simulink model "KALTITUDE_V1"  (R2015b)
settings: Solver=ode2  StartTime=0.0  StopTime=65  FixedStep=0.01  RelTol=1e-3
undefined symbols (not defined in the file or in its folder): sigbuilder_block
settings Model: SimulationMode=accelerator  Creator=asus  LastModifiedBy=asus

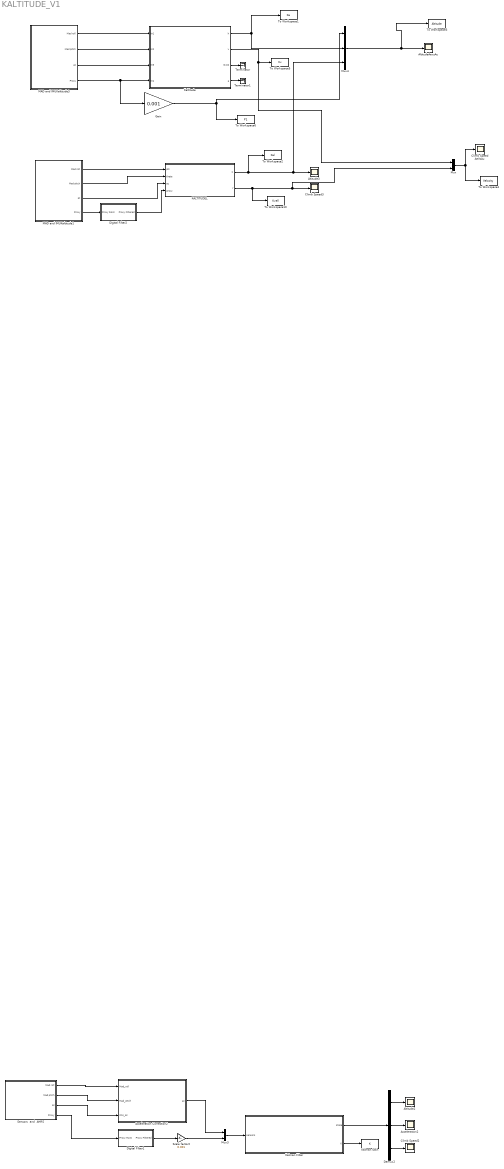
== system KALTITUDE_V1 ==
  Acceleration Correction2 : MATLAB Function  TreatAsAtomicUnit=on
  Acceleration2 : Scope
  Altitude2 : Scope
  Altitude3 : Scope
  AltitudeAevsAu : Scope
  Climb Speed AeVsAu : Scope
  Climb Speed2 : Scope
  Climb Speed3 : Scope
  Demux2 : Demux  Outputs=[1 1 1]
  Digital Filter1 : Subsystem
  Digital Filter2 : Subsystem
  Gain : Gain  Gain=0.001
  KALTITUDEL : Subsystem
  Kalman Filter : Subsystem
  Kalman Gain : ToWorkspace  VariableName=K  SaveFormat=Timeseries  SampleTime=-1
  Kaltitude : Subsystem
  MAD and IMUKaltitude1 : Subsystem
  MAD and IMUKaltitude3 : Subsystem
  Mux : Mux  Inputs=[1 1]
  Mux3 : Mux  Inputs=2
  Mux4 : Mux  Inputs=[1 1 1]
  Scale factor2 : Gain  Gain=0.001
  "Sensors  and  AHRS " : Subsystem
  Terminator : Terminator
  Terminator1 : Terminator
  To Workspace1 : ToWorkspace  VariableName=Ka  SampleTime=-1
  To Workspace10 : ToWorkspace  VariableName=Kvell  SampleTime=-1
  To Workspace2 : ToWorkspace  VariableName=Kal  SampleTime=-1
  To Workspace3 : ToWorkspace  VariableName=Altitude  SampleTime=-1
  To Workspace4 : ToWorkspace  VariableName=Velocity  SampleTime=-1
  To Workspace5 : ToWorkspace  VariableName=Kv  SampleTime=-1
  To Workspace6 : ToWorkspace  VariableName=P1  SampleTime=-1
  wires:
  Kalman Filter/1(state) -> Demux2/1
  Kalman Filter/2(K) -> Kalman Gain/1
  Mux3/1 -> Kalman Filter/1(sensors)
  Demux2/1 -> Altitude2/1
  Demux2/3 -> Climb Speed2/1
  Demux2/2 -> Acceleration2/1
  Scale factor2/1 -> Mux3/2
  Acceleration Correction2/1(az) -> Mux3/1
  "Sensors  and  AHRS "/1(Mad roll) -> Acceleration Correction2/1(Mad_roll)
  "Sensors  and  AHRS "/2(Mad pitch) -> Acceleration Correction2/2(Mad_pitch)
  "Sensors  and  AHRS "/3(az) -> Acceleration Correction2/3(IMU_az)
  "Sensors  and  AHRS "/4(Proxy) -> Digital Filter1/1(Proxy RAW)
  Digital Filter1/1(Proxy Filtered) -> Scale factor2/1
  MAD and IMUKaltitude1/4(Proxy) -> Digital Filter2/1(Proxy RAW)
  Digital Filter2/1(Proxy Filtered) -> KALTITUDEL/4(proxy)
  MAD and IMUKaltitude1/3(az) -> KALTITUDEL/3(az)
  MAD and IMUKaltitude1/2(Mad pitch) -> KALTITUDEL/2(theta)
  MAD and IMUKaltitude1/1(Mad roll) -> KALTITUDEL/1(phi)
  Mux/1 -> To Workspace4/1, Climb Speed AeVsAu/1
  Mux4/1 -> To Workspace3/1, AltitudeAevsAu/1
  MAD and IMUKaltitude3/1(Mad roll) -> Kaltitude/1(In1)
  MAD and IMUKaltitude3/2(Mad pitch) -> Kaltitude/2(In2)
  MAD and IMUKaltitude3/3(az) -> Kaltitude/3(In3)
  MAD and IMUKaltitude3/4(Proxy) -> Gain/1, Kaltitude/4(In4)
  KALTITUDEL/1(h) -> To Workspace2/1, Mux4/3, Altitude3/1
  KALTITUDEL/2(v) -> To Workspace10/1, Mux/2, Climb Speed3/1
  Kaltitude/1(h) -> Mux4/2, To Workspace1/1
  Kaltitude/2(v) -> To Workspace5/1, Mux/1
  Gain/1 -> Mux4/1, To Workspace6/1
  Kaltitude/3(Out2) -> Terminator/1
  Kaltitude/4(a) -> Terminator1/1

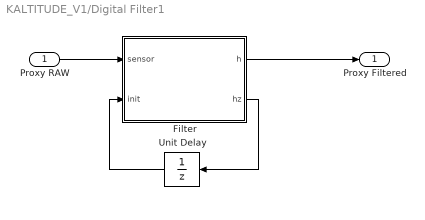
== system KALTITUDE_V1/Digital Filter1 ==
  Proxy RAW : Inport
  Filter : MATLAB Function  TreatAsAtomicUnit=on
  Unit Delay : UnitDelay  SampleTime=-1
  Proxy Filtered : Outport
  wires:
  Filter/2(hz) -> Unit Delay/1
  Unit Delay/1 -> Filter/2(init)
  Proxy RAW/1 -> Filter/1(sensor)
  Filter/1(h) -> Proxy Filtered/1

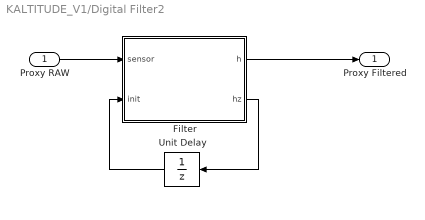
== system KALTITUDE_V1/Digital Filter2 ==
  Proxy RAW : Inport
  Filter : MATLAB Function  TreatAsAtomicUnit=on
  Unit Delay : UnitDelay  SampleTime=-1
  Proxy Filtered : Outport
  wires:
  Filter/1(h) -> Proxy Filtered/1
  Proxy RAW/1 -> Filter/1(sensor)
  Unit Delay/1 -> Filter/2(init)
  Filter/2(hz) -> Unit Delay/1

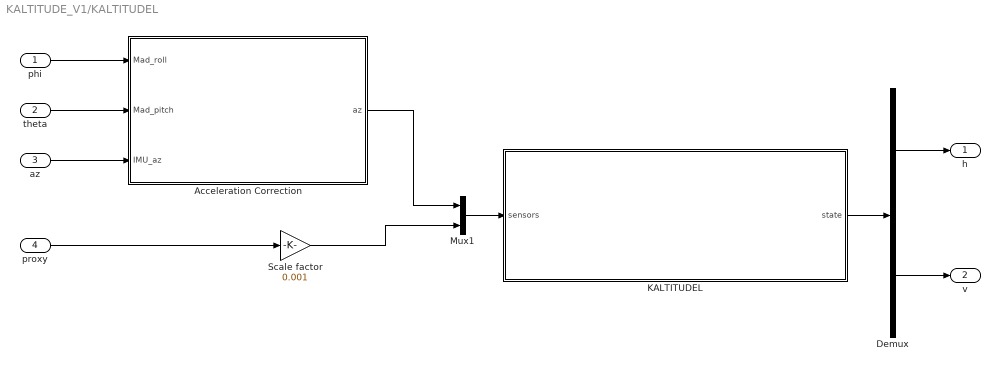
== system KALTITUDE_V1/KALTITUDEL ==
  phi : Inport
  theta : Inport  Port=2
  az : Inport  Port=3
  proxy : Inport  Port=4
  Acceleration Correction : MATLAB Function  TreatAsAtomicUnit=on
  Demux : Demux  Outputs=2
  KALTITUDEL : Subsystem
  Mux1 : Mux  Inputs=2
  Scale factor : Gain  Gain=0.001
  h : Outport
  v : Outport  Port=2
  wires:
  Acceleration Correction/1(az) -> Mux1/1
  Scale factor/1 -> Mux1/2
  proxy/1 -> Scale factor/1
  Mux1/1 -> KALTITUDEL/1(sensors)
  theta/1 -> Acceleration Correction/2(Mad_pitch)
  phi/1 -> Acceleration Correction/1(Mad_roll)
  az/1 -> Acceleration Correction/3(IMU_az)
  KALTITUDEL/1(state) -> Demux/1
  Demux/1 -> h/1
  Demux/2 -> v/1

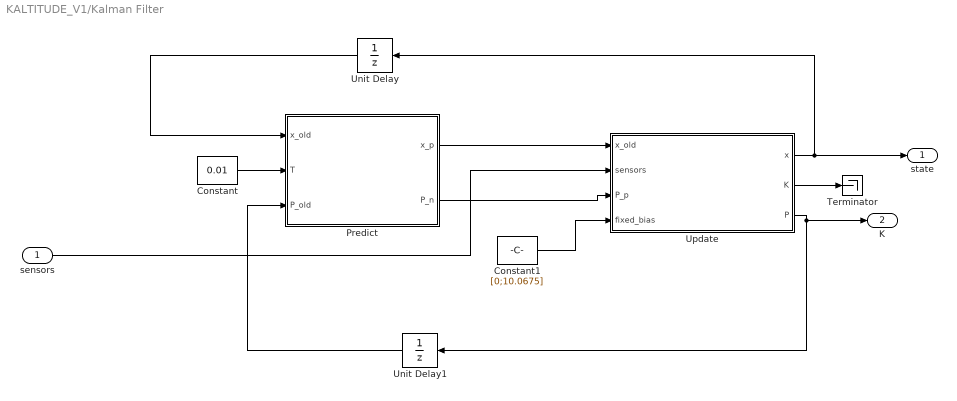
== system KALTITUDE_V1/Kalman Filter ==
  sensors : Inport
  Constant : Constant  Value=0.01  VectorParams1D=off  SampleTime=-1
  Constant1 : Constant  Value=[0;10.0675]  VectorParams1D=off  SampleTime=-1
  "Predict " : MATLAB Function  TreatAsAtomicUnit=on
  Terminator : Terminator
  Unit Delay : UnitDelay  InitialCondition=zeros(3,1)  SampleTime=-1
  Unit Delay1 : UnitDelay  InitialCondition=eye(3)*0.001  SampleTime=-1
  Update : MATLAB Function  TreatAsAtomicUnit=on
  state : Outport
  K : Outport  Port=2
  wires:
  Update/2(K) -> Terminator/1
  Unit Delay1/1 -> "Predict "/3(P_old)
  Update/1(x) -> state/1, Unit Delay/1
  "Predict "/1(x_p) -> Update/1(x_old)
  Constant1/1 -> Update/4(fixed_bias)
  sensors/1 -> Update/2(sensors)
  "Predict "/2(P_n) -> Update/3(P_p)
  Constant/1 -> "Predict "/2(T)
  Update/3(P) -> Unit Delay1/1, K/1
  Unit Delay/1 -> "Predict "/1(x_old)

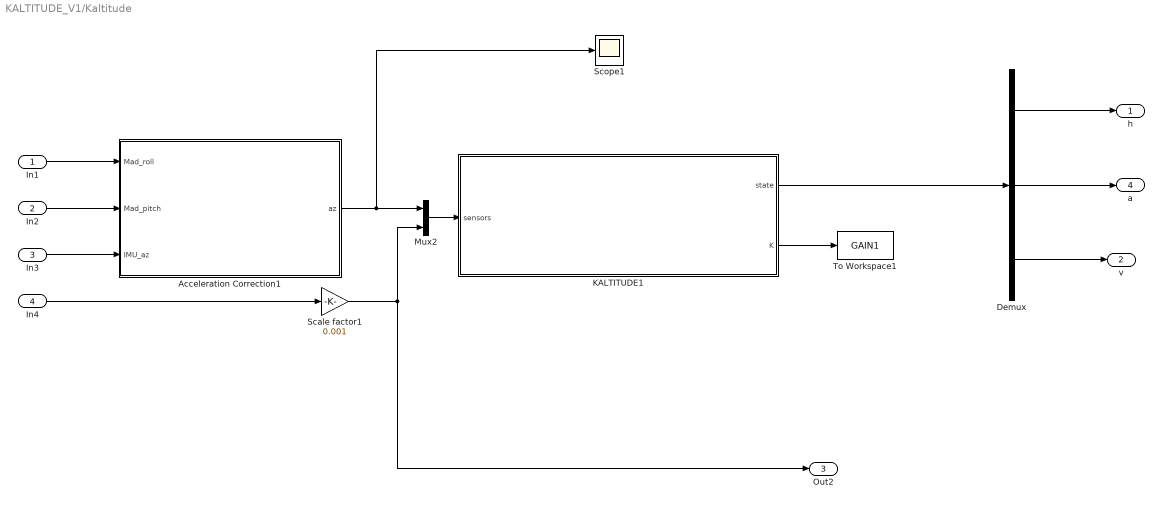
== system KALTITUDE_V1/Kaltitude ==
  In1 : Inport
  In2 : Inport  Port=2
  In3 : Inport  Port=3
  In4 : Inport  Port=4
  Acceleration Correction1 : MATLAB Function  TreatAsAtomicUnit=on
  Demux : Demux  Outputs=3
  KALTITUDE1 : Subsystem
  Mux2 : Mux  Inputs=2
  Scale factor1 : Gain  Gain=0.001
  Scope1 : Scope
  To Workspace1 : ToWorkspace  VariableName=GAIN1  SaveFormat=Timeseries  SampleTime=-1
  h : Outport
  v : Outport  Port=2
  Out2 : Outport  Port=3
  a : Outport  Port=4
  wires:
  Mux2/1 -> KALTITUDE1/1(sensors)
  KALTITUDE1/2(K) -> To Workspace1/1
  Acceleration Correction1/1(az) -> Mux2/1, Scope1/1
  In3/1 -> Acceleration Correction1/3(IMU_az)
  In4/1 -> Scale factor1/1
  In1/1 -> Acceleration Correction1/1(Mad_roll)
  In2/1 -> Acceleration Correction1/2(Mad_pitch)
  Scale factor1/1 -> Out2/1, Mux2/2
  KALTITUDE1/1(state) -> Demux/1
  Demux/1 -> h/1
  Demux/2 -> a/1
  Demux/3 -> v/1

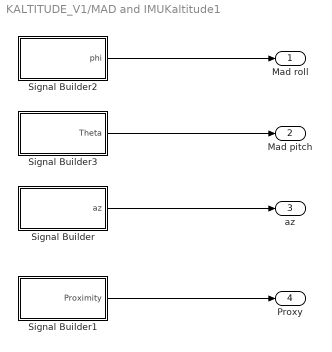
== system KALTITUDE_V1/MAD and IMUKaltitude1 ==
  Signal Builder : Subsystem  Tag=STV Subsys  LoadFcn=sigbuilder_block('load');  StartFcn=sigbuilder_block('start');  StopFcn=sigbuilder_block('stop');  ClipboardFcn=sigbuilder_block('clipboard');  mask(Sigbuilder block){}
      mask init:
      | if ~strcmp(get_param(bdroot(gcb),'SimulationStatus'),'stopped'),tuvar = sigbuilder_block('maskInit'); end
      settings: CopyFcn=sigbuilder_block('copy');  DeleteFcn=sigbuilder_block('delete');  ModelCloseFcn=sigbuilder_block('modelClose');  PreSaveFcn=sigbuilder_block('preSave');  PauseFcn=sigbuilder_block('pause');  ContinueFcn=sigbuilder_block('continue');  NameChangeFcn=sigbuilder_block('namechange');  OpenFcn=sigbuilder_block('open',[50 50 520 400 ]);  CloseFcn=sigbuilder_block('close');
      mask Display: plot(0, 0, 100, 100,[2, 2, 32, 32, 2], [68, 8, 8, 68, 68],[32, 2], [38, 38], [32, 19, 2],[53, 60, 44], [32, 17, 17, 2],[16, 16, 31, 31]);txt = getActiveGroup(gcbh);text(2, 100, txt,'verticalAlignment', 'top');
  Signal Builder1 : Subsystem  Tag=STV Subsys  LoadFcn=sigbuilder_block('load');  StartFcn=sigbuilder_block('start');  StopFcn=sigbuilder_block('stop');  ClipboardFcn=sigbuilder_block('clipboard');  mask(Sigbuilder block){}
      mask init:
      | if ~strcmp(get_param(bdroot(gcb),'SimulationStatus'),'stopped'),tuvar = sigbuilder_block('maskInit'); end
      settings: CopyFcn=sigbuilder_block('copy');  DeleteFcn=sigbuilder_block('delete');  ModelCloseFcn=sigbuilder_block('modelClose');  PreSaveFcn=sigbuilder_block('preSave');  PauseFcn=sigbuilder_block('pause');  ContinueFcn=sigbuilder_block('continue');  NameChangeFcn=sigbuilder_block('namechange');  OpenFcn=sigbuilder_block('open');  CloseFcn=sigbuilder_block('close');
      mask Display: plot(0, 0, 100, 100,[2, 2, 32, 32, 2], [68, 8, 8, 68, 68],[32, 2], [38, 38], [32, 19, 2],[53, 60, 44], [32, 17, 17, 2],[16, 16, 31, 31]);txt = getActiveGroup(gcbh);text(2, 100, txt,'verticalAlignment', 'top');
  Signal Builder2 : Subsystem  Tag=STV Subsys  LoadFcn=sigbuilder_block('load');  StartFcn=sigbuilder_block('start');  StopFcn=sigbuilder_block('stop');  ClipboardFcn=sigbuilder_block('clipboard');  mask(Sigbuilder block){}
      mask init:
      | if ~strcmp(get_param(bdroot(gcb),'SimulationStatus'),'stopped'),tuvar = sigbuilder_block('maskInit'); end
      settings: CopyFcn=sigbuilder_block('copy');  DeleteFcn=sigbuilder_block('delete');  ModelCloseFcn=sigbuilder_block('modelClose');  PreSaveFcn=sigbuilder_block('preSave');  PauseFcn=sigbuilder_block('pause');  ContinueFcn=sigbuilder_block('continue');  NameChangeFcn=sigbuilder_block('namechange');  OpenFcn=sigbuilder_block('open');  CloseFcn=sigbuilder_block('close');
      mask Display: plot(0, 0, 100, 100,[2, 2, 32, 32, 2], [68, 8, 8, 68, 68],[32, 2], [38, 38], [32, 19, 2],[53, 60, 44], [32, 17, 17, 2],[16, 16, 31, 31]);txt = getActiveGroup(gcbh);text(2, 100, txt,'verticalAlignment', 'top');
  Signal Builder3 : Subsystem  Tag=STV Subsys  LoadFcn=sigbuilder_block('load');  StartFcn=sigbuilder_block('start');  StopFcn=sigbuilder_block('stop');  ClipboardFcn=sigbuilder_block('clipboard');  mask(Sigbuilder block){}
      mask init:
      | if ~strcmp(get_param(bdroot(gcb),'SimulationStatus'),'stopped'),tuvar = sigbuilder_block('maskInit'); end
      settings: CopyFcn=sigbuilder_block('copy');  DeleteFcn=sigbuilder_block('delete');  ModelCloseFcn=sigbuilder_block('modelClose');  PreSaveFcn=sigbuilder_block('preSave');  PauseFcn=sigbuilder_block('pause');  ContinueFcn=sigbuilder_block('continue');  NameChangeFcn=sigbuilder_block('namechange');  OpenFcn=sigbuilder_block('open');  CloseFcn=sigbuilder_block('close');
      mask Display: plot(0, 0, 100, 100,[2, 2, 32, 32, 2], [68, 8, 8, 68, 68],[32, 2], [38, 38], [32, 19, 2],[53, 60, 44], [32, 17, 17, 2],[16, 16, 31, 31]);txt = getActiveGroup(gcbh);text(2, 100, txt,'verticalAlignment', 'top');
  Mad roll : Outport
  Mad pitch : Outport  Port=2
  az : Outport  Port=3
  Proxy : Outport  Port=4
  wires:
  Signal Builder3/1(Theta) -> Mad pitch/1
  Signal Builder/1(az) -> az/1
  Signal Builder1/1(Proximity) -> Proxy/1
  Signal Builder2/1(phi) -> Mad roll/1

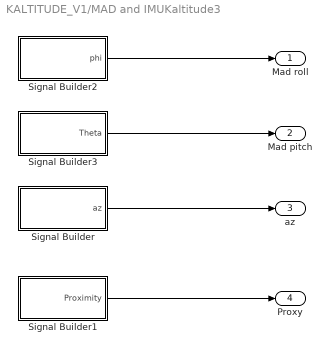
== system KALTITUDE_V1/MAD and IMUKaltitude3 ==
  Signal Builder : Subsystem  Tag=STV Subsys  LoadFcn=sigbuilder_block('load');  StartFcn=sigbuilder_block('start');  StopFcn=sigbuilder_block('stop');  ClipboardFcn=sigbuilder_block('clipboard');  mask(Sigbuilder block){}
      mask init:
      | if ~strcmp(get_param(bdroot(gcb),'SimulationStatus'),'stopped'),tuvar = sigbuilder_block('maskInit'); end
      settings: CopyFcn=sigbuilder_block('copy');  DeleteFcn=sigbuilder_block('delete');  ModelCloseFcn=sigbuilder_block('modelClose');  PreSaveFcn=sigbuilder_block('preSave');  PauseFcn=sigbuilder_block('pause');  ContinueFcn=sigbuilder_block('continue');  NameChangeFcn=sigbuilder_block('namechange');  OpenFcn=sigbuilder_block('open',[50 50 520 400 ]);  CloseFcn=sigbuilder_block('close');
      mask Display: plot(0, 0, 100, 100,[2, 2, 32, 32, 2], [68, 8, 8, 68, 68],[32, 2], [38, 38], [32, 19, 2],[53, 60, 44], [32, 17, 17, 2],[16, 16, 31, 31]);txt = getActiveGroup(gcbh);text(2, 100, txt,'verticalAlignment', 'top');
  Signal Builder1 : Subsystem  Tag=STV Subsys  LoadFcn=sigbuilder_block('load');  StartFcn=sigbuilder_block('start');  StopFcn=sigbuilder_block('stop');  ClipboardFcn=sigbuilder_block('clipboard');  mask(Sigbuilder block){}
      mask init:
      | if ~strcmp(get_param(bdroot(gcb),'SimulationStatus'),'stopped'),tuvar = sigbuilder_block('maskInit'); end
      settings: CopyFcn=sigbuilder_block('copy');  DeleteFcn=sigbuilder_block('delete');  ModelCloseFcn=sigbuilder_block('modelClose');  PreSaveFcn=sigbuilder_block('preSave');  PauseFcn=sigbuilder_block('pause');  ContinueFcn=sigbuilder_block('continue');  NameChangeFcn=sigbuilder_block('namechange');  OpenFcn=sigbuilder_block('open');  CloseFcn=sigbuilder_block('close');
      mask Display: plot(0, 0, 100, 100,[2, 2, 32, 32, 2], [68, 8, 8, 68, 68],[32, 2], [38, 38], [32, 19, 2],[53, 60, 44], [32, 17, 17, 2],[16, 16, 31, 31]);txt = getActiveGroup(gcbh);text(2, 100, txt,'verticalAlignment', 'top');
  Signal Builder2 : Subsystem  Tag=STV Subsys  LoadFcn=sigbuilder_block('load');  StartFcn=sigbuilder_block('start');  StopFcn=sigbuilder_block('stop');  ClipboardFcn=sigbuilder_block('clipboard');  mask(Sigbuilder block){}
      mask init:
      | if ~strcmp(get_param(bdroot(gcb),'SimulationStatus'),'stopped'),tuvar = sigbuilder_block('maskInit'); end
      settings: CopyFcn=sigbuilder_block('copy');  DeleteFcn=sigbuilder_block('delete');  ModelCloseFcn=sigbuilder_block('modelClose');  PreSaveFcn=sigbuilder_block('preSave');  PauseFcn=sigbuilder_block('pause');  ContinueFcn=sigbuilder_block('continue');  NameChangeFcn=sigbuilder_block('namechange');  OpenFcn=sigbuilder_block('open');  CloseFcn=sigbuilder_block('close');
      mask Display: plot(0, 0, 100, 100,[2, 2, 32, 32, 2], [68, 8, 8, 68, 68],[32, 2], [38, 38], [32, 19, 2],[53, 60, 44], [32, 17, 17, 2],[16, 16, 31, 31]);txt = getActiveGroup(gcbh);text(2, 100, txt,'verticalAlignment', 'top');
  Signal Builder3 : Subsystem  Tag=STV Subsys  LoadFcn=sigbuilder_block('load');  StartFcn=sigbuilder_block('start');  StopFcn=sigbuilder_block('stop');  ClipboardFcn=sigbuilder_block('clipboard');  mask(Sigbuilder block){}
      mask init:
      | if ~strcmp(get_param(bdroot(gcb),'SimulationStatus'),'stopped'),tuvar = sigbuilder_block('maskInit'); end
      settings: CopyFcn=sigbuilder_block('copy');  DeleteFcn=sigbuilder_block('delete');  ModelCloseFcn=sigbuilder_block('modelClose');  PreSaveFcn=sigbuilder_block('preSave');  PauseFcn=sigbuilder_block('pause');  ContinueFcn=sigbuilder_block('continue');  NameChangeFcn=sigbuilder_block('namechange');  OpenFcn=sigbuilder_block('open');  CloseFcn=sigbuilder_block('close');
      mask Display: plot(0, 0, 100, 100,[2, 2, 32, 32, 2], [68, 8, 8, 68, 68],[32, 2], [38, 38], [32, 19, 2],[53, 60, 44], [32, 17, 17, 2],[16, 16, 31, 31]);txt = getActiveGroup(gcbh);text(2, 100, txt,'verticalAlignment', 'top');
  Mad roll : Outport
  Mad pitch : Outport  Port=2
  az : Outport  Port=3
  Proxy : Outport  Port=4
  wires:
  Signal Builder2/1(phi) -> Mad roll/1
  Signal Builder1/1(Proximity) -> Proxy/1
  Signal Builder/1(az) -> az/1
  Signal Builder3/1(Theta) -> Mad pitch/1

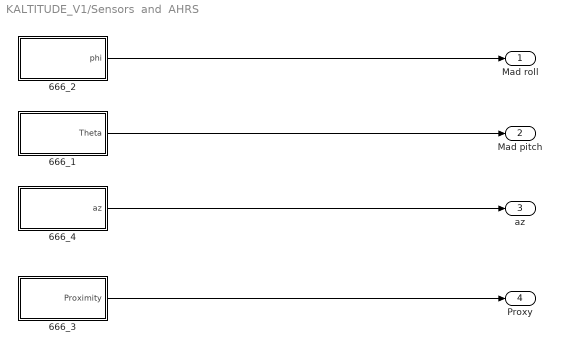
== system KALTITUDE_V1/Sensors  and  AHRS  ==
  666_1 : Subsystem  Tag=STV Subsys  LoadFcn=sigbuilder_block('load');  StartFcn=sigbuilder_block('start');  StopFcn=sigbuilder_block('stop');  ClipboardFcn=sigbuilder_block('clipboard');  mask(Sigbuilder block){}
      mask init:
      | if ~strcmp(get_param(bdroot(gcb),'SimulationStatus'),'stopped'),tuvar = sigbuilder_block('maskInit'); end
      settings: CopyFcn=sigbuilder_block('copy');  DeleteFcn=sigbuilder_block('delete');  ModelCloseFcn=sigbuilder_block('modelClose');  PreSaveFcn=sigbuilder_block('preSave');  PauseFcn=sigbuilder_block('pause');  ContinueFcn=sigbuilder_block('continue');  NameChangeFcn=sigbuilder_block('namechange');  OpenFcn=sigbuilder_block('open');  CloseFcn=sigbuilder_block('close');
      mask Display: plot(0, 0, 100, 100,[2, 2, 32, 32, 2], [68, 8, 8, 68, 68],[32, 2], [38, 38], [32, 19, 2],[53, 60, 44], [32, 17, 17, 2],[16, 16, 31, 31]);txt = getActiveGroup(gcbh);text(2, 100, txt,'verticalAlignment', 'top');
  666_2 : Subsystem  Tag=STV Subsys  LoadFcn=sigbuilder_block('load');  StartFcn=sigbuilder_block('start');  StopFcn=sigbuilder_block('stop');  ClipboardFcn=sigbuilder_block('clipboard');  mask(Sigbuilder block){}
      mask init:
      | if ~strcmp(get_param(bdroot(gcb),'SimulationStatus'),'stopped'),tuvar = sigbuilder_block('maskInit'); end
      settings: CopyFcn=sigbuilder_block('copy');  DeleteFcn=sigbuilder_block('delete');  ModelCloseFcn=sigbuilder_block('modelClose');  PreSaveFcn=sigbuilder_block('preSave');  PauseFcn=sigbuilder_block('pause');  ContinueFcn=sigbuilder_block('continue');  NameChangeFcn=sigbuilder_block('namechange');  OpenFcn=sigbuilder_block('open');  CloseFcn=sigbuilder_block('close');
      mask Display: plot(0, 0, 100, 100,[2, 2, 32, 32, 2], [68, 8, 8, 68, 68],[32, 2], [38, 38], [32, 19, 2],[53, 60, 44], [32, 17, 17, 2],[16, 16, 31, 31]);txt = getActiveGroup(gcbh);text(2, 100, txt,'verticalAlignment', 'top');
  666_3 : Subsystem  Tag=STV Subsys  LoadFcn=sigbuilder_block('load');  StartFcn=sigbuilder_block('start');  StopFcn=sigbuilder_block('stop');  ClipboardFcn=sigbuilder_block('clipboard');  mask(Sigbuilder block){}
      mask init:
      | if ~strcmp(get_param(bdroot(gcb),'SimulationStatus'),'stopped'),tuvar = sigbuilder_block('maskInit'); end
      settings: CopyFcn=sigbuilder_block('copy');  DeleteFcn=sigbuilder_block('delete');  ModelCloseFcn=sigbuilder_block('modelClose');  PreSaveFcn=sigbuilder_block('preSave');  PauseFcn=sigbuilder_block('pause');  ContinueFcn=sigbuilder_block('continue');  NameChangeFcn=sigbuilder_block('namechange');  OpenFcn=sigbuilder_block('open');  CloseFcn=sigbuilder_block('close');
      mask Display: plot(0, 0, 100, 100,[2, 2, 32, 32, 2], [68, 8, 8, 68, 68],[32, 2], [38, 38], [32, 19, 2],[53, 60, 44], [32, 17, 17, 2],[16, 16, 31, 31]);txt = getActiveGroup(gcbh);text(2, 100, txt,'verticalAlignment', 'top');
  666_4 : Subsystem  Tag=STV Subsys  LoadFcn=sigbuilder_block('load');  StartFcn=sigbuilder_block('start');  StopFcn=sigbuilder_block('stop');  ClipboardFcn=sigbuilder_block('clipboard');  mask(Sigbuilder block){}
      mask init:
      | if ~strcmp(get_param(bdroot(gcb),'SimulationStatus'),'stopped'),tuvar = sigbuilder_block('maskInit'); end
      settings: CopyFcn=sigbuilder_block('copy');  DeleteFcn=sigbuilder_block('delete');  ModelCloseFcn=sigbuilder_block('modelClose');  PreSaveFcn=sigbuilder_block('preSave');  PauseFcn=sigbuilder_block('pause');  ContinueFcn=sigbuilder_block('continue');  NameChangeFcn=sigbuilder_block('namechange');  OpenFcn=sigbuilder_block('open');  CloseFcn=sigbuilder_block('close');
      mask Display: plot(0, 0, 100, 100,[2, 2, 32, 32, 2], [68, 8, 8, 68, 68],[32, 2], [38, 38], [32, 19, 2],[53, 60, 44], [32, 17, 17, 2],[16, 16, 31, 31]);txt = getActiveGroup(gcbh);text(2, 100, txt,'verticalAlignment', 'top');
  Mad roll : Outport
  Mad pitch : Outport  Port=2
  az : Outport  Port=3
  Proxy : Outport  Port=4
  wires:
  666_2/1(phi) -> Mad roll/1
  666_3/1(Proximity) -> Proxy/1
  666_4/1(az) -> az/1
  666_1/1(Theta) -> Mad pitch/1

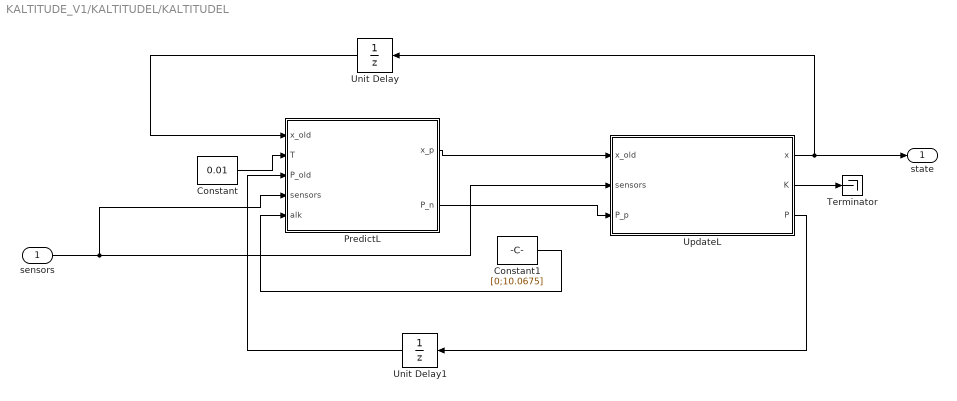
== system KALTITUDE_V1/KALTITUDEL/KALTITUDEL ==
  sensors : Inport
  Constant : Constant  Value=0.01  VectorParams1D=off  SampleTime=-1
  Constant1 : Constant  Value=[0;10.0675]  VectorParams1D=off  SampleTime=-1
  "PredictL " : MATLAB Function  TreatAsAtomicUnit=on
  Terminator : Terminator
  Unit Delay : UnitDelay  InitialCondition=zeros(2,1)  SampleTime=-1
  Unit Delay1 : UnitDelay  InitialCondition=eye(2)*0.001  SampleTime=-1
  UpdateL : MATLAB Function  TreatAsAtomicUnit=on
  state : Outport
  wires:
  Unit Delay/1 -> "PredictL "/1(x_old)
  UpdateL/3(P) -> Unit Delay1/1
  Constant/1 -> "PredictL "/2(T)
  "PredictL "/2(P_n) -> UpdateL/3(P_p)
  Constant1/1 -> "PredictL "/5(alk)
  "PredictL "/1(x_p) -> UpdateL/1(x_old)
  UpdateL/1(x) -> Unit Delay/1, state/1
  Unit Delay1/1 -> "PredictL "/3(P_old)
  UpdateL/2(K) -> Terminator/1
  sensors/1 -> UpdateL/2(sensors), "PredictL "/4(sensors)

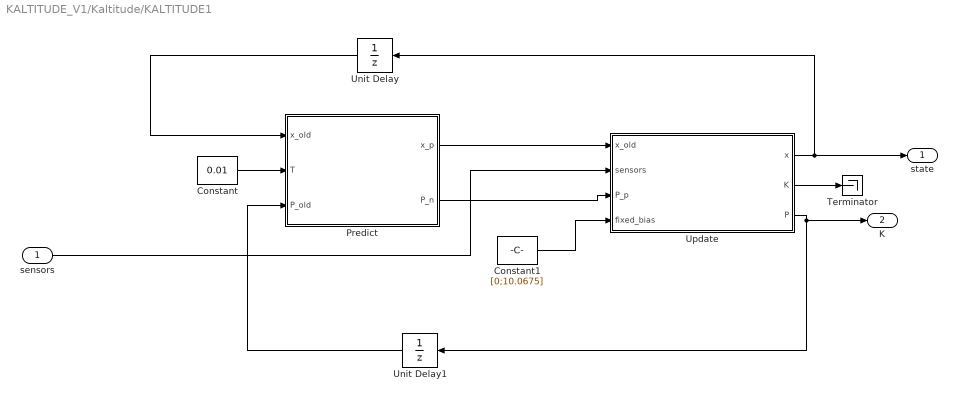
== system KALTITUDE_V1/Kaltitude/KALTITUDE1 ==
  sensors : Inport
  Constant : Constant  Value=0.01  VectorParams1D=off  SampleTime=-1
  Constant1 : Constant  Value=[0;10.0675]  VectorParams1D=off  SampleTime=-1
  "Predict " : MATLAB Function  TreatAsAtomicUnit=on
  Terminator : Terminator
  Unit Delay : UnitDelay  InitialCondition=zeros(3,1)  SampleTime=-1
  Unit Delay1 : UnitDelay  InitialCondition=eye(3)*0.001  SampleTime=-1
  Update : MATLAB Function  TreatAsAtomicUnit=on
  state : Outport
  K : Outport  Port=2
  wires:
  Update/2(K) -> Terminator/1
  Unit Delay1/1 -> "Predict "/3(P_old)
  Update/1(x) -> state/1, Unit Delay/1
  "Predict "/1(x_p) -> Update/1(x_old)
  Constant1/1 -> Update/4(fixed_bias)
  sensors/1 -> Update/2(sensors)
  "Predict "/2(P_n) -> Update/3(P_p)
  Constant/1 -> "Predict "/2(T)
  Update/3(P) -> Unit Delay1/1, K/1
  Unit Delay/1 -> "Predict "/1(x_old)

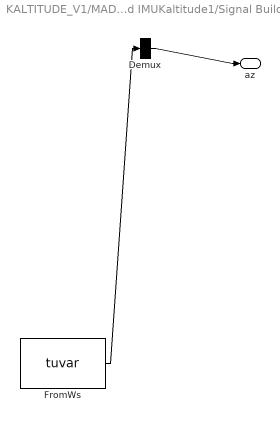
== system KALTITUDE_V1/MAD and IMUKaltitude1/Signal Builder ==
  Demux : Demux  Tag=STV Demux  Outputs=1
  FromWs : FromWorkspace  Tag=STV FromWs  VariableName=tuvar  SampleTime=0
      SigBuilderData=|
      | dataSet.timeRange = [0 78.28]
      | dataSet.name = 'Group 1'
      | sbobj.Name = 'Signal Builder'
      | sbobj.Groups.Name = 'Group 1'
      | sbobj.Groups.Signals.Name = 'az'
      | sbobj.Groups.Signals.XData = [0 0.01 0.02 0.03 0.04 0.05 0.06 0.07 0.08 0.09 0.1 0.11 ... (7829 elements, 1x7829)]
      | sbobj.Groups.Signals.YData = [10.1200966 10.0009198 10.0605082 10.1101652 9.981057 10.0505768 10.0108512 9.9909884 10.0505768 10.0207826 10.080371 10.0605082 ... (7829 elements, 1x7829)]
      | sbobj.Groups.TimeRange = [0 78.28]
  az : Outport  Tag=STV Outport
  wires:
  FromWs/1 -> Demux/1
  Demux/1 -> az/1

== system KALTITUDE_V1/MAD and IMUKaltitude1/Signal Builder1 ==
  Demux : Demux  Tag=STV Demux  Outputs=1
  FromWs : FromWorkspace  Tag=STV FromWs  VariableName=tuvar  SampleTime=0
      SigBuilderData=|
      | dataSet.timeRange = [0 78.28]
      | dataSet.name = 'Group 1'
      | sbobj.Name = 'Signal Builder'
      | sbobj.Groups.Name = 'Group 1'
      | sbobj.Groups.Signals.Name = 'Proximity'
      | sbobj.Groups.Signals.XData = [0 0.01 0.02 0.03 0.04 0.05 0.06 0.07 0.08 0.09 0.1 0.11 ... (7829 elements, 1x7829)]
      | sbobj.Groups.Signals.YData = [263 263 263 263 263 263 263 263 263 263 263 263 ... (7829 elements, 1x7829)]
      | sbobj.Groups.TimeRange = [0 78.28]
  Proximity : Outport  Tag=STV Outport
  wires:
  FromWs/1 -> Demux/1
  Demux/1 -> Proximity/1

== system KALTITUDE_V1/MAD and IMUKaltitude1/Signal Builder2 ==
  Demux : Demux  Tag=STV Demux  Outputs=1
  FromWs : FromWorkspace  Tag=STV FromWs  VariableName=tuvar  SampleTime=0
      SigBuilderData=|
      | dataSet.timeRange = [0 78.28]
      | dataSet.name = 'Group 1'
      | sbobj.Name = 'Signal Builder'
      | sbobj.Groups.Name = 'Group 1'
      | sbobj.Groups.Signals.Name = 'phi'
      | sbobj.Groups.Signals.XData = [0 0.01 0.02 0.03 0.04 0.05 0.06 0.07 0.08 0.09 0.1 0.11 ... (7829 elements, 1x7829)]
      | sbobj.Groups.Signals.YData = [-0.015331 -0.015021 -0.015246 -0.015383 -0.015158 -0.015836 -0.01575 -0.015446 -0.015278 -0.01489 -0.015048 -0.015493 ... (7829 elements, 1x7829)]
      | sbobj.Groups.TimeRange = [0 78.28]
  phi : Outport  Tag=STV Outport
  wires:
  FromWs/1 -> Demux/1
  Demux/1 -> phi/1

== system KALTITUDE_V1/MAD and IMUKaltitude1/Signal Builder3 ==
  Demux : Demux  Tag=STV Demux  Outputs=1
  FromWs : FromWorkspace  Tag=STV FromWs  VariableName=tuvar  SampleTime=0
      SigBuilderData=|
      | dataSet.timeRange = [0 78.28]
      | dataSet.name = 'Group 1'
      | sbobj.Name = 'Signal Builder'
      | sbobj.Groups.Name = 'Group 1'
      | sbobj.Groups.Signals.Name = 'Theta'
      | sbobj.Groups.Signals.XData = [0 0.01 0.02 0.03 0.04 0.05 0.06 0.07 0.08 0.09 0.1 0.11 ... (7829 elements, 1x7829)]
      | sbobj.Groups.Signals.YData = [0.003862 0.004183 0.00458 0.004215 0.004584 0.004601 0.004884 0.004487 0.004301 0.004059 0.003732 0.003878 ... (7829 elements, 1x7829)]
      | sbobj.Groups.TimeRange = [0 78.28]
  Theta : Outport  Tag=STV Outport
  wires:
  FromWs/1 -> Demux/1
  Demux/1 -> Theta/1

== system KALTITUDE_V1/MAD and IMUKaltitude3/Signal Builder ==
  Demux : Demux  Tag=STV Demux  Outputs=1
  FromWs : FromWorkspace  Tag=STV FromWs  VariableName=tuvar  SampleTime=0
      SigBuilderData=|
      | dataSet.timeRange = [0 78.28]
      | dataSet.name = 'Group 1'
      | sbobj.Name = 'Signal Builder'
      | sbobj.Groups.Name = 'Group 1'
      | sbobj.Groups.Signals.Name = 'az'
      | sbobj.Groups.Signals.XData = [0 0.01 0.02 0.03 0.04 0.05 0.06 0.07 0.08 0.09 0.1 0.11 ... (7829 elements, 1x7829)]
      | sbobj.Groups.Signals.YData = [10.1200966 10.0009198 10.0605082 10.1101652 9.981057 10.0505768 10.0108512 9.9909884 10.0505768 10.0207826 10.080371 10.0605082 ... (7829 elements, 1x7829)]
      | sbobj.Groups.TimeRange = [0 78.28]
  az : Outport  Tag=STV Outport
  wires:
  Demux/1 -> az/1
  FromWs/1 -> Demux/1

== system KALTITUDE_V1/MAD and IMUKaltitude3/Signal Builder1 ==
  Demux : Demux  Tag=STV Demux  Outputs=1
  FromWs : FromWorkspace  Tag=STV FromWs  VariableName=tuvar  SampleTime=0
      SigBuilderData=|
      | dataSet.timeRange = [0 78.28]
      | dataSet.name = 'Group 1'
      | sbobj.Name = 'Signal Builder'
      | sbobj.Groups.Name = 'Group 1'
      | sbobj.Groups.Signals.Name = 'Proximity'
      | sbobj.Groups.Signals.XData = [0 0.01 0.02 0.03 0.04 0.05 0.06 0.07 0.08 0.09 0.1 0.11 ... (7829 elements, 1x7829)]
      | sbobj.Groups.Signals.YData = [263 263 263 263 263 263 263 263 263 263 263 263 ... (7829 elements, 1x7829)]
      | sbobj.Groups.TimeRange = [0 78.28]
  Proximity : Outport  Tag=STV Outport
  wires:
  Demux/1 -> Proximity/1
  FromWs/1 -> Demux/1

== system KALTITUDE_V1/MAD and IMUKaltitude3/Signal Builder2 ==
  Demux : Demux  Tag=STV Demux  Outputs=1
  FromWs : FromWorkspace  Tag=STV FromWs  VariableName=tuvar  SampleTime=0
      SigBuilderData=|
      | dataSet.timeRange = [0 78.28]
      | dataSet.name = 'Group 1'
      | sbobj.Name = 'Signal Builder'
      | sbobj.Groups.Name = 'Group 1'
      | sbobj.Groups.Signals.Name = 'phi'
      | sbobj.Groups.Signals.XData = [0 0.01 0.02 0.03 0.04 0.05 0.06 0.07 0.08 0.09 0.1 0.11 ... (7829 elements, 1x7829)]
      | sbobj.Groups.Signals.YData = [-0.015331 -0.015021 -0.015246 -0.015383 -0.015158 -0.015836 -0.01575 -0.015446 -0.015278 -0.01489 -0.015048 -0.015493 ... (7829 elements, 1x7829)]
      | sbobj.Groups.TimeRange = [0 78.28]
  phi : Outport  Tag=STV Outport
  wires:
  Demux/1 -> phi/1
  FromWs/1 -> Demux/1

== system KALTITUDE_V1/MAD and IMUKaltitude3/Signal Builder3 ==
  Demux : Demux  Tag=STV Demux  Outputs=1
  FromWs : FromWorkspace  Tag=STV FromWs  VariableName=tuvar  SampleTime=0
      SigBuilderData=|
      | dataSet.timeRange = [0 78.28]
      | dataSet.name = 'Group 1'
      | sbobj.Name = 'Signal Builder'
      | sbobj.Groups.Name = 'Group 1'
      | sbobj.Groups.Signals.Name = 'Theta'
      | sbobj.Groups.Signals.XData = [0 0.01 0.02 0.03 0.04 0.05 0.06 0.07 0.08 0.09 0.1 0.11 ... (7829 elements, 1x7829)]
      | sbobj.Groups.Signals.YData = [0.003862 0.004183 0.00458 0.004215 0.004584 0.004601 0.004884 0.004487 0.004301 0.004059 0.003732 0.003878 ... (7829 elements, 1x7829)]
      | sbobj.Groups.TimeRange = [0 78.28]
  Theta : Outport  Tag=STV Outport
  wires:
  Demux/1 -> Theta/1
  FromWs/1 -> Demux/1

== system KALTITUDE_V1/Sensors  and  AHRS /666_1 ==
  Demux : Demux  Tag=STV Demux  Outputs=1
  FromWs : FromWorkspace  Tag=STV FromWs  VariableName=tuvar  SampleTime=0
      SigBuilderData=|
      | dataSet.timeRange = [0 28.78]
      | dataSet.name = 'Group 1'
      | sbobj.Name = 'Signal Builder'
      | sbobj.Groups.Name = 'Group 1'
      | sbobj.Groups.Signals.Name = 'Theta'
      | sbobj.Groups.Signals.XData = [0 0.01 0.02 0.03 0.04 0.05 0.06 0.07 0.08 0.09 0.1 0.11 ... (2879 elements, 1x2879)]
      | sbobj.Groups.Signals.YData = [0.0096771700239 0.00941994339874 0.00991804291397 0.00981747704247 0.00990996203953 0.00947457220433 0.0104326357906 0.0103889676527 0.0110546187762 0.0102572651074 0.0108417933272 0.0101831933339 ... (2879 elements, 1x2879)]
      | sbobj.Groups.TimeRange = [0 28.78]
  Theta : Outport  Tag=STV Outport
  wires:
  Demux/1 -> Theta/1
  FromWs/1 -> Demux/1

== system KALTITUDE_V1/Sensors  and  AHRS /666_2 ==
  Demux : Demux  Tag=STV Demux  Outputs=1
  FromWs : FromWorkspace  Tag=STV FromWs  VariableName=tuvar  SampleTime=0
      SigBuilderData=|
      | dataSet.timeRange = [0 28.78]
      | dataSet.name = 'Group 1'
      | sbobj.Name = 'Signal Builder'
      | sbobj.Groups.Name = 'Group 1'
      | sbobj.Groups.Signals.Name = 'phi'
      | sbobj.Groups.Signals.XData = [0 0.01 0.02 0.03 0.04 0.05 0.06 0.07 0.08 0.09 0.1 0.11 ... (2879 elements, 1x2879)]
      | sbobj.Groups.Signals.YData = [-0.00931187261146 -0.00897631560947 -0.00909025070304 -0.00966798959203 -0.00923195398501 -0.00927426076608 -0.00966179367319 -0.00968266781104 -0.00928799650729 -0.00964598099017 -0.00914187754231 -0.00914442572302 ... (2879 elements, 1x2879)]
      | sbobj.Groups.TimeRange = [0 28.78]
  phi : Outport  Tag=STV Outport
  wires:
  Demux/1 -> phi/1
  FromWs/1 -> Demux/1

== system KALTITUDE_V1/Sensors  and  AHRS /666_3 ==
  Demux : Demux  Tag=STV Demux  Outputs=1
  FromWs : FromWorkspace  Tag=STV FromWs  VariableName=tuvar  SampleTime=0
      SigBuilderData=|
      | dataSet.timeRange = [0 28.78]
      | dataSet.name = 'Group 1'
      | sbobj.Name = 'Signal Builder'
      | sbobj.Groups.Name = 'Group 1'
      | sbobj.Groups.Signals.Name = 'Proximity'
      | sbobj.Groups.Signals.XData = [0 0.01 0.02 0.03 0.04 0.05 0.06 0.07 0.08 0.09 0.1 0.11 ... (2879 elements, 1x2879)]
      | sbobj.Groups.Signals.YData = [0 0 0 0 0 0 0 0 0 0 0 0 ... (2879 elements, 1x2879)]
      | sbobj.Groups.TimeRange = [0 28.78]
  Proximity : Outport  Tag=STV Outport
  wires:
  Demux/1 -> Proximity/1
  FromWs/1 -> Demux/1

== system KALTITUDE_V1/Sensors  and  AHRS /666_4 ==
  Demux : Demux  Tag=STV Demux  Outputs=1
  FromWs : FromWorkspace  Tag=STV FromWs  VariableName=tuvar  SampleTime=0
      SigBuilderData=|
      | dataSet.timeRange = [0 28.78]
      | dataSet.name = 'Group 1'
      | sbobj.Name = 'Signal Builder'
      | sbobj.Groups.Name = 'Group 1'
      | sbobj.Groups.Signals.Name = 'az'
      | sbobj.Groups.Signals.XData = [0 0.01 0.02 0.03 0.04 0.05 0.06 0.07 0.08 0.09 0.1 0.11 ... (2879 elements, 1x2879)]
      | sbobj.Groups.Signals.YData = [10.1598222 10.1399594 10.1697536 10.1598222 10.130028 10.1498908 10.130028 10.1498908 10.1995478 10.1598222 10.1598222 10.1598222 ... (2879 elements, 1x2879)]
      | sbobj.Groups.TimeRange = [0 28.78]
  az : Outport  Tag=STV Outport
  wires:
  Demux/1 -> az/1
  FromWs/1 -> Demux/1

== matlab function KALTITUDE_V1/Kaltitude/Acceleration Correction1 ==
  data: Mad_roll input; az output; Mad_pitch input; IMU_az input
function az = Accelerometer_correction(Mad_roll,Mad_pitch,IMU_az)
%#codegen
az = (IMU_az/10.06-sqrt(1-(sin(Mad_roll)^2+sin(Mad_pitch)^2)))*9.81;

== matlab function KALTITUDE_V1/Digital Filter1/Filter ==
  data: sensor input; h output; init input; hz output
%% Filtro 2 %%
%%%%%%%%%%%%%%

function [h,hz] = filter(sensor,init)
hz = init;
if(sensor<=161 || sensor>=5000)
    h = hz;
else if(abs(sensor-hz)>=300)
        h = hz;
    else
        hz = sensor;
        h = hz;
    end
end

== matlab function KALTITUDE_V1/Kaltitude/KALTITUDE1/Predict  ==
  data x_old settings: description=State estimate at the previous step.
  data x_p settings: description=A-priori state estimate.
  data T settings: description=Control signal at the previous step.
  data P_n settings: description=A-priori covariance estimate.
  data P_old settings: description=Covariance estimate at the previous step.
  data: x_old input; x_p output; T input; P_n output; P_old input
%%EKF  state update       %
% Author: Matteo Ferronato%
% Last review: 2016/02/09 %
%%%%%%%%%%%%%%%%%%%%%%%%%%%
%% Description
% The purpose of this script is to calculate the state update of
% Extended Kalman Filter 
%%
function [x_p,P_n] = state_update(x_old,T,P_old)


Qn = eye(3)*0.005;
% Qn(1,1)=3;
% Qn(2,2)=0.01;
%% Initialize variables

A = [ 1, T^2/2, T;
      0,   1,   0;
      0,   T,   1];

x_p = A*x_old;   

%% Jacobian initialization
 P_n = A*P_old*A' + Qn;

== matlab function KALTITUDE_V1/Kaltitude/KALTITUDE1/Update ==
  data x_old settings: description=A-priori state estimate.
  data sensors settings: description=Measurements from the sensors.
  data x settings: description=Corrected state estimate.
  data P_p settings: description=A-priori covariance estimate.
  data P settings: description=Corrected covariance estimate.
  data: x_old input; sensors input; x output; K output; P_p input; P output; fixed_bias input
%%EKF  state correction       %
% Author: Matteo Ferronato%
% Last review: 2016/02/09 %
%%%%%%%%%%%%%%%%%%%%%%%%%%%
%% Description
% The purpose of this script is to calculate the state update of
% Extended Kalman Filter 
%%
function [x,K,P] = state_correction(x_old,sensors,P_p,fixed_bias)

% Useful Parameters

sigma = 0.71485;
Rn = eye(2)*1*sigma;
Rn(2,2) = 1; 

alk= fixed_bias(2);
sensors(1,1) = (sensors(1,1));



%%
H = [0 1 0;
     1 0 0];
     
 %%
   h = H*x_old;
        
%%
Pl = P_p; 
x_p = x_old;

for j = 1:2
% Innovation covariance
S = H(j,:)*Pl*H(j,:)' + Rn(j,j);

% Kalman gain
K = Pl*H(j,:)'/S;

% Updated state estimate
x_p = x_p + K*(sensors(j,1)-h(j,1));

% Updated estimated covariance
Pl = (eye(3) - K*H(j,:))*Pl*(eye(3) - K*H(j,:))' + K*Rn(j,j)*K';
end

P = Pl;
x = x_p;

== matlab function KALTITUDE_V1/Acceleration Correction2 ==
  data: Mad_roll input; az output; Mad_pitch input; IMU_az input
function az = Accelerometer_correction(Mad_roll,Mad_pitch,IMU_az)
%#codegen
az =(IMU_az/norm(IMU_az) + sqrt(1-sin(Mad_roll)^2+sin(Mad_pitch)^2))*9.81;

== matlab function KALTITUDE_V1/Kalman Filter/Predict  ==
  data x_old settings: description=State estimate at the previous step.
  data x_p settings: description=A-priori state estimate.
  data T settings: description=Control signal at the previous step.
  data P_n settings: description=A-priori covariance estimate.
  data P_old settings: description=Covariance estimate at the previous step.
  data: x_old input; x_p output; T input; P_n output; P_old input
%%EKF  state update       %
% Author: Matteo Ferronato%
% Last review: 2016/02/09 %
%%%%%%%%%%%%%%%%%%%%%%%%%%%
%% Description
% The purpose of this script is to calculate the state update of
% Extended Kalman Filter 
%%
function [x_p,P_n] = state_update(x_old,T,P_old)


Qn = eye(3)*0.001;
% Qn(1,1)=3;
% Qn(2,2)=0.01;
%% Initialize variables

A = [ 1, T^2/2, T;
      0,   1,   0;
      0,   T,   1];

x_p = A*x_old;   

%% Jacobian initialization
 P_n = A*P_old*A' + Qn;

== matlab function KALTITUDE_V1/Kalman Filter/Update ==
  data x_old settings: description=A-priori state estimate.
  data sensors settings: description=Measurements from the sensors.
  data x settings: description=Corrected state estimate.
  data P_p settings: description=A-priori covariance estimate.
  data P settings: description=Corrected covariance estimate.
  data: x_old input; sensors input; x output; K output; P_p input; P output; fixed_bias input
%%EKF  state correction       %
% Author: Matteo Ferronato%
% Last review: 2016/02/09 %
%%%%%%%%%%%%%%%%%%%%%%%%%%%
%% Description
% The purpose of this script is to calculate the state update of
% Extended Kalman Filter 
%%
function [x,K,P] = state_correction(x_old,sensors,P_p,fixed_bias)

% Useful Parameters


Rn = eye(2)*0.0012;
Rn(2,2) = 0.001; 

alk= fixed_bias(2);
sensors(1,1) = 9.81*(sensors(1,1) - alk/norm(alk));



%%
H = [0 1 0;
     1 0 0];
     
 %%
   h = H*x_old;
        
%%
Pl = P_p; 
x_p = x_old;

for j = 1:2
% Innovation covariance
S = H(j,:)*Pl*H(j,:)' + Rn(j,j);

% Kalman gain
K = Pl*H(j,:)'/S;

% Updated state estimate
x_p = x_p + K*(sensors(j,1)-h(j,1));

% Updated estimated covariance
Pl = (eye(3) - K*H(j,:))*Pl*(eye(3) - K*H(j,:))' + K*Rn(j,j)*K';
end

P = Pl;
x = x_p;

== matlab function KALTITUDE_V1/KALTITUDEL/Acceleration Correction ==
  data: Mad_roll input; az output; Mad_pitch input; IMU_az input
function az = Accelerometer_correction(Mad_roll,Mad_pitch,IMU_az)
%#codegen
az = (IMU_az/10.06-sqrt(1-(sin(Mad_roll)^2+sin(Mad_pitch)^2)))*10.06;

== matlab function KALTITUDE_V1/KALTITUDEL/KALTITUDEL/PredictL  ==
  data x_old settings: description=State estimate at the previous step.
  data x_p settings: description=A-priori state estimate.
  data T settings: description=Control signal at the previous step.
  data P_n settings: description=A-priori covariance estimate.
  data P_old settings: description=Covariance estimate at the previous step.
  data: x_old input; x_p output; T input; P_n output; P_old input; sensors input; alk input
%%EKF  state update       %
% Author: Matteo Ferronato%
% Last review: 2016/02/09 %
%%%%%%%%%%%%%%%%%%%%%%%%%%%
%% Description
% The purpose of this script is to calculate the state update of
% Extended Kalman Filter 
%%
function [x_p,P_n] = state_update(x_old,T,P_old,sensors,alk)

u = sensors(1);

Qn = zeros(2,2);
% Qn(1,1)=3;
Qn(2,2)=0.71485;
%% Initialize variables

A = [ 1,  T;
      0,  1];
  
G = [T^2/2;
     T];

x_p = A*x_old + G*u;

%% Jacobian initialization
 P_n = A*P_old*A' + G*Qn(2,2)*G';

== matlab function KALTITUDE_V1/KALTITUDEL/KALTITUDEL/UpdateL ==
  data x_old settings: description=A-priori state estimate.
  data sensors settings: description=Measurements from the sensors.
  data x settings: description=Corrected state estimate.
  data P_p settings: description=A-priori covariance estimate.
  data P settings: description=Corrected covariance estimate.
  data: x_old input; sensors input; x output; K output; P_p input; P output
%%EKF  state correction       %
% Author: Matteo Ferronato%
% Last review: 2016/02/09 %
%%%%%%%%%%%%%%%%%%%%%%%%%%%
%% Description
% The purpose of this script is to calculate the state update of
% Extended Kalman Filter 
%%
function [x,K,P] = state_correction(x_old,sensors,P_p)

% Useful Parameters


Rn = 0.01;




%%
H = [1 0];
     
 %%
   h = H*x_old;
        
%%
Pl = P_p; 
x_p = x_old;


% Innovation covariance
S = H*Pl*H' + Rn;

% Kalman gain
K = Pl*H'/S;

% Updated state estimate
x_p = x_p + K*(sensors(2)-h);

% Updated estimated covariance
Pl = (eye(2) - K*H)*Pl*(eye(2) - K*H)' + K*Rn*K';


P = Pl;
x = x_p;

== matlab function KALTITUDE_V1/Digital Filter2/Filter ==
  data: sensor input; h output; init input; hz output
%% Filtro 2 %%
%%%%%%%%%%%%%%

function [h,hz] = filter(sensor,init)
hz = init;
if(sensor<=161 || sensor>=5000)
    h = hz;
else if(abs(sensor-hz)>=300)
        h = hz;
    else
        hz = sensor;
        h = hz;
    end
end
